simulink subsystem "sm_inbound_interpreter"  (R2023a)
settings: Solver=VariableStepAuto  StartTime=0.0  StopTime=10.0  RelTol=1e-3
undefined symbols (not defined in the file or in its folder): ARMED, AUX1, AUX2, AUX3, AUX4, AUX5, AUX6, EXTR1, EXTR2, EXTR3, EXTR4, EXTR5, EXTR6, MODE, Pitch, Roll, Throttle, Yaw
settings Model: Creator=gcs_comp1  LastModifiedBy=thesa

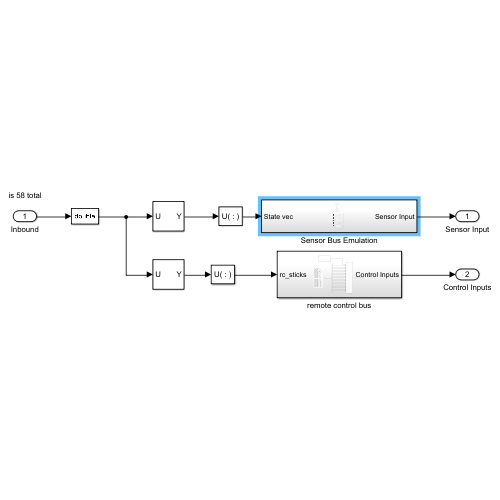
[thumbnail: Simulink's stored preview of the top-level diagram]
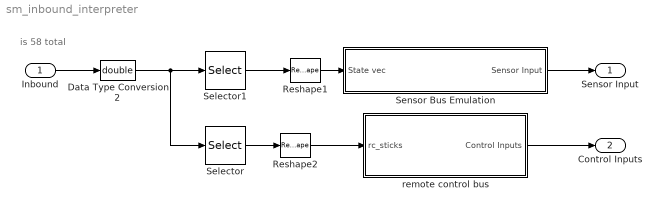
== system sm_inbound_interpreter ==
  note: is 58 total
  Inbound : Inport
  Data Type Conversion2 : DataTypeConversion  OutDataTypeStr=double  SaturateOnIntegerOverflow=off  RndMeth=Floor
  Reshape1 : Reshape
  Reshape2 : Reshape
  Selector : Selector  InputPortWidth=58  IndexOptions=Index vector (dialog)  Indices=[1:18]  OutputSizes=1
  Selector1 : Selector  InputPortWidth=58  IndexOptions=Index vector (dialog)  Indices=[(1:40) + 18]  OutputSizes=1
  Sensor Bus Emulation : Subsystem
  remote control bus : Subsystem
  Sensor Input : Outport
  Control Inputs : Outport  Port=2
  wires:
  Sensor Bus Emulation/1(Sensor Input) -> Sensor Input/1
  remote control bus/1(Control Inputs) -> Control Inputs/1
  Reshape2/1 -> remote control bus/1(rc_sticks)
  Reshape1/1 -> Sensor Bus Emulation/1(State vec)
  Selector/1 -> Reshape2/1
  Selector1/1 -> Reshape1/1
  Data Type Conversion2/1 -> Selector1/1, Selector/1
  Inbound/1 -> Data Type Conversion2/1

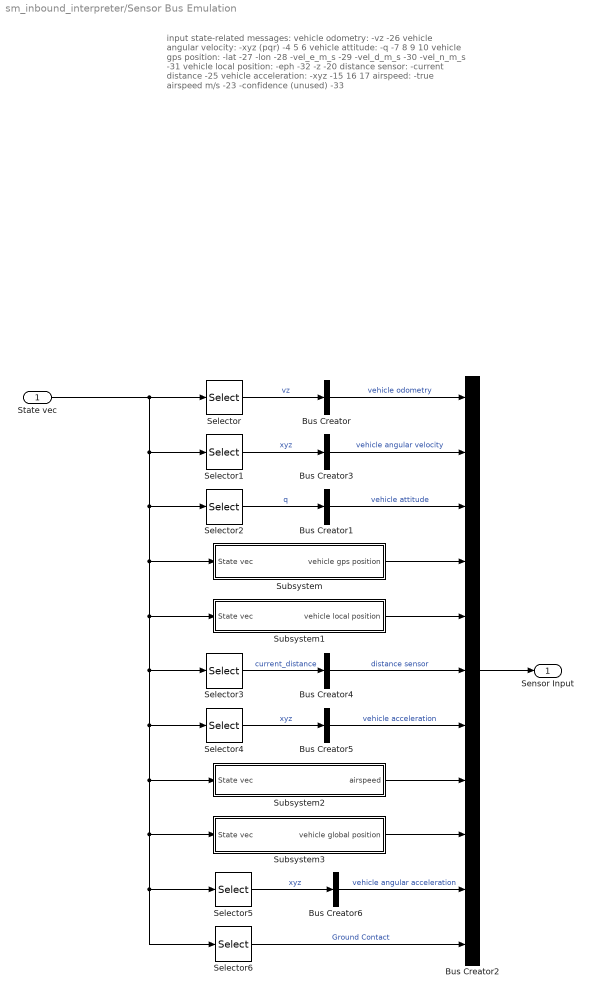
== system sm_inbound_interpreter/Sensor Bus Emulation ==
  note: input state-related messages:
      | vehicle odometry:
      | -vz -26
      | vehicle angular velocity:
      | -xyz (pqr) -4 5 6
      | vehicle attitude:
      | -q -7 8 9 10
      | vehicle gps position:
      | -lat -27
      | -lon -28
      | -vel_e_m_s -29
      | -vel_d_m_s -30
      | -vel_n_m_s -31
      | vehicle local position:
      | -eph -32
      | -z -20
      | distance sensor:
      | -current distance -25
      | vehicle acceleration:
      | -xyz -15 16 17
      | airspeed:
      | -true airspeed m/s -23
      | -confidence (unused) -33
  State vec : Inport
  Bus Creator{,1,3..6} (6 alike) : BusCreator  Inputs=1
  Bus Creator2 : BusCreator  Inputs=11
  Selector : Selector  InputPortWidth=40  IndexOptions=Index vector (dialog)  Indices=[26]  OutputSizes=1
  Selector1 : Selector  InputPortWidth=40  IndexOptions=Index vector (dialog)  Indices=[4 5 6]  OutputSizes=1
  Selector2 : Selector  InputPortWidth=40  IndexOptions=Index vector (dialog)  Indices=[7 8 9 10]  OutputSizes=1
  Selector3 : Selector  InputPortWidth=40  IndexOptions=Index vector (dialog)  Indices=[25]  OutputSizes=1
  Selector4 : Selector  InputPortWidth=40  IndexOptions=Index vector (dialog)  Indices=[15 16 17]  OutputSizes=1
  Selector5 : Selector  InputPortWidth=40  IndexOptions=Index vector (dialog)  Indices=[34:36]  OutputSizes=1
  Selector6 : Selector  InputPortWidth=40  IndexOptions=Index vector (dialog)  Indices=[22]  OutputSizes=1
  Subsystem : Subsystem
  Subsystem1 : Subsystem
  Subsystem2 : Subsystem
  Subsystem3 : Subsystem
  Sensor Input : Outport
  wires:
  Selector6/1 -> Bus Creator2/11  "Ground Contact"
  Subsystem3/1(vehicle global position) -> Bus Creator2/9
  Subsystem2/1(airspeed) -> Bus Creator2/8
  Bus Creator5/1 -> Bus Creator2/7  "vehicle acceleration"
  Selector4/1 -> Bus Creator5/1  "xyz"
  Bus Creator4/1 -> Bus Creator2/6  "distance sensor"
  Selector3/1 -> Bus Creator4/1  "current_distance"
  Subsystem1/1(vehicle local position) -> Bus Creator2/5
  Subsystem/1(vehicle gps position) -> Bus Creator2/4
  Bus Creator1/1 -> Bus Creator2/3  "vehicle attitude"
  Selector2/1 -> Bus Creator1/1  "q"
  Bus Creator2/1 -> Sensor Input/1
  Bus Creator/1 -> Bus Creator2/1  "vehicle odometry"
  Bus Creator3/1 -> Bus Creator2/2  "vehicle angular velocity"
  Selector/1 -> Bus Creator/1  "vz"
  Selector1/1 -> Bus Creator3/1  "xyz"
  Selector5/1 -> Bus Creator6/1  "xyz"
  State vec/1 -> Selector/1, Selector1/1, Selector2/1, Subsystem/1(State vec), Subsystem1/1(State vec), Selector3/1, Selector4/1, Subsystem2/1(State vec), Selector5/1, Selector6/1, Subsystem3/1(State vec)
  Bus Creator6/1 -> Bus Creator2/10  "vehicle angular acceleration"

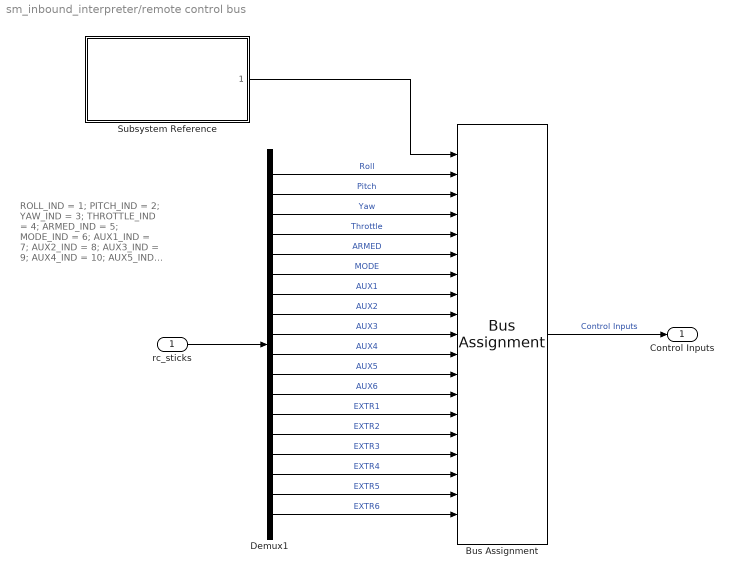
== system sm_inbound_interpreter/remote control bus ==
  note: ROLL_IND = 1;
      | PITCH_IND = 2;
      | YAW_IND = 3;
      | THROTTLE_IND = 4;
      | ARMED_IND = 5;
      | MODE_IND = 6;
      | AUX1_IND = 7;
      | AUX2_IND = 8;
      | AUX3_IND = 9;
      | AUX4_IND = 10;
      | AUX5_IND = 11;
      | AUX6_IND = 12;
      | EXTR1_IND = 13;
      | EXTR2_IND = 14;
      | EXTR3_IND = 15;
      | EXTR4_IND = 16;
      | EXTR5_IND = 17;
      | EXTR6_IND = 18;
  rc_sticks : Inport
  Bus Assignment : BusAssignment  AssignedSignals=Roll,Pitch,Yaw,Throttle,ARMED,MODE,AUX1,AUX2,AUX3,AUX4,AUX5,AUX6,EXTR1,EXTR2,EXTR3,EXTR4,EXTR5,EXTR6
  Demux1 : Demux  Outputs=18
  Subsystem Reference : Subsystem  ReferencedSubsystem=sm_rc_initializer
  Control Inputs : Outport
  wires:
  Demux1/17 -> Bus Assignment/18  "EXTR5"
  Demux1/18 -> Bus Assignment/19  "EXTR6"
  Demux1/16 -> Bus Assignment/17  "EXTR4"
  Demux1/15 -> Bus Assignment/16  "EXTR3"
  Demux1/14 -> Bus Assignment/15  "EXTR2"
  Demux1/13 -> Bus Assignment/14  "EXTR1"
  Demux1/12 -> Bus Assignment/13  "AUX6"
  Demux1/11 -> Bus Assignment/12  "AUX5"
  Demux1/10 -> Bus Assignment/11  "AUX4"
  Demux1/9 -> Bus Assignment/10  "AUX3"
  Demux1/8 -> Bus Assignment/9  "AUX2"
  Demux1/7 -> Bus Assignment/8  "AUX1"
  Demux1/6 -> Bus Assignment/7  "MODE"
  Demux1/5 -> Bus Assignment/6  "ARMED"
  Demux1/4 -> Bus Assignment/5  "Throttle"
  Demux1/3 -> Bus Assignment/4  "Yaw"
  rc_sticks/1 -> Demux1/1
  Bus Assignment/1 -> Control Inputs/1  "Control Inputs"
  Demux1/2 -> Bus Assignment/3  "Pitch"
  Demux1/1 -> Bus Assignment/2  "Roll"
  Subsystem Reference/1 -> Bus Assignment/1

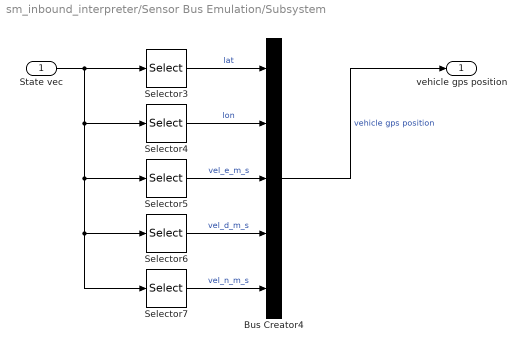
== system sm_inbound_interpreter/Sensor Bus Emulation/Subsystem ==
  State vec : Inport
  Bus Creator4 : BusCreator  Inputs=5
  Selector3 : Selector  InputPortWidth=40  IndexOptions=Index vector (dialog)  Indices=[27]  OutputSizes=1
  Selector4 : Selector  InputPortWidth=40  IndexOptions=Index vector (dialog)  Indices=[28]  OutputSizes=1
  Selector5 : Selector  InputPortWidth=40  IndexOptions=Index vector (dialog)  Indices=[29]  OutputSizes=1
  Selector6 : Selector  InputPortWidth=40  IndexOptions=Index vector (dialog)  Indices=[30]  OutputSizes=1
  Selector7 : Selector  InputPortWidth=40  IndexOptions=Index vector (dialog)  Indices=[31]  OutputSizes=1
  vehicle gps position : Outport
  wires:
  Bus Creator4/1 -> vehicle gps position/1  "vehicle gps position"
  Selector3/1 -> Bus Creator4/1  "lat"
  Selector6/1 -> Bus Creator4/4  "vel_d_m_s"
  Selector4/1 -> Bus Creator4/2  "lon"
  Selector7/1 -> Bus Creator4/5  "vel_n_m_s"
  State vec/1 -> Selector4/1, Selector5/1, Selector7/1, Selector6/1, Selector3/1
  Selector5/1 -> Bus Creator4/3  "vel_e_m_s"

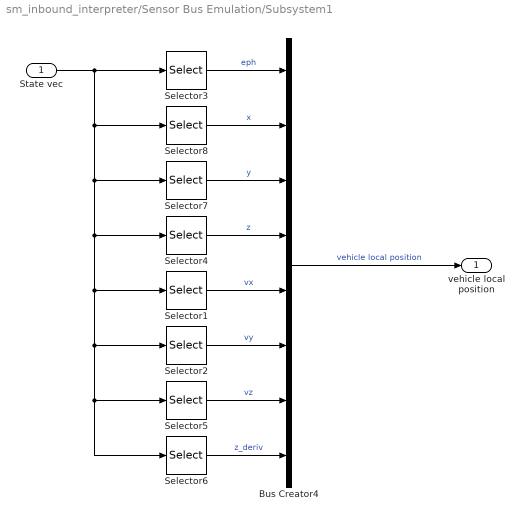
== system sm_inbound_interpreter/Sensor Bus Emulation/Subsystem1 ==
  State vec : Inport
  Bus Creator4 : BusCreator  Inputs=8
  Selector1 : Selector  InputPortWidth=40  IndexOptions=Index vector (dialog)  Indices=[1]  OutputSizes=1
  Selector2 : Selector  InputPortWidth=40  IndexOptions=Index vector (dialog)  Indices=[2]  OutputSizes=1
  Selector3 : Selector  InputPortWidth=40  IndexOptions=Index vector (dialog)  Indices=[32]  OutputSizes=1
  Selector4 : Selector  InputPortWidth=40  IndexOptions=Index vector (dialog)  Indices=[20]  OutputSizes=1
  Selector5 : Selector  InputPortWidth=40  IndexOptions=Index vector (dialog)  Indices=[3]  OutputSizes=1
  Selector6 : Selector  InputPortWidth=40  IndexOptions=Index vector (dialog)  Indices=[21]  OutputSizes=1
  Selector7 : Selector  InputPortWidth=40  IndexOptions=Index vector (dialog)  Indices=[19]  OutputSizes=1
  Selector8 : Selector  InputPortWidth=40  IndexOptions=Index vector (dialog)  Indices=[18]  OutputSizes=1
  vehicle local position : Outport
  wires:
  Selector6/1 -> Bus Creator4/8  "z_deriv"
  Selector7/1 -> Bus Creator4/3  "y"
  Selector8/1 -> Bus Creator4/2  "x"
  Selector5/1 -> Bus Creator4/7  "vz"
  Selector2/1 -> Bus Creator4/6  "vy"
  Selector1/1 -> Bus Creator4/5  "vx"
  State vec/1 -> Selector3/1, Selector8/1, Selector1/1, Selector5/1, Selector6/1, Selector2/1, Selector4/1, Selector7/1
  Selector4/1 -> Bus Creator4/4  "z"
  Selector3/1 -> Bus Creator4/1  "eph"
  Bus Creator4/1 -> vehicle local position/1  "vehicle local position"

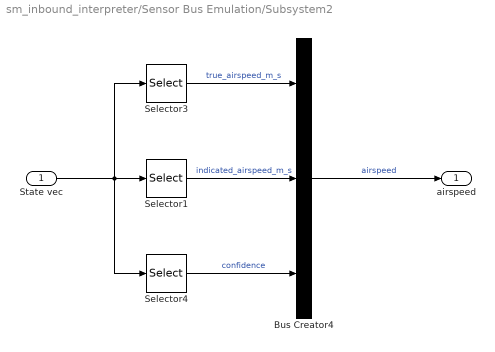
== system sm_inbound_interpreter/Sensor Bus Emulation/Subsystem2 ==
  State vec : Inport
  Bus Creator4 : BusCreator  Inputs=3
  Selector1 : Selector  InputPortWidth=40  IndexOptions=Index vector (dialog)  Indices=[24]  OutputSizes=1
  Selector3 : Selector  InputPortWidth=40  IndexOptions=Index vector (dialog)  Indices=[23]  OutputSizes=1
  Selector4 : Selector  InputPortWidth=40  IndexOptions=Index vector (dialog)  Indices=[33]  OutputSizes=1
  airspeed : Outport
  wires:
  Selector1/1 -> Bus Creator4/2  "indicated_airspeed_m_s"
  Bus Creator4/1 -> airspeed/1  "airspeed"
  Selector3/1 -> Bus Creator4/1  "true_airspeed_m_s"
  Selector4/1 -> Bus Creator4/3  "confidence"
  State vec/1 -> Selector4/1, Selector1/1, Selector3/1

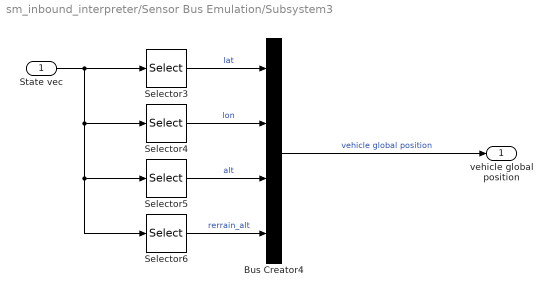
== system sm_inbound_interpreter/Sensor Bus Emulation/Subsystem3 ==
  State vec : Inport
  Bus Creator4 : BusCreator  Inputs=4
  Selector3 : Selector  InputPortWidth=40  IndexOptions=Index vector (dialog)  Indices=[11]  OutputSizes=1
  Selector4 : Selector  InputPortWidth=40  IndexOptions=Index vector (dialog)  Indices=[12]  OutputSizes=1
  Selector5 : Selector  InputPortWidth=40  IndexOptions=Index vector (dialog)  Indices=[13]  OutputSizes=1
  Selector6 : Selector  InputPortWidth=40  IndexOptions=Index vector (dialog)  Indices=[14]  OutputSizes=1
  vehicle global position : Outport
  wires:
  Selector5/1 -> Bus Creator4/3  "alt"
  State vec/1 -> Selector3/1, Selector6/1, Selector5/1, Selector4/1
  Selector4/1 -> Bus Creator4/2  "lon"
  Selector6/1 -> Bus Creator4/4  "rerrain_alt"
  Selector3/1 -> Bus Creator4/1  "lat"
  Bus Creator4/1 -> vehicle global position/1  "vehicle global position"
